simulink model "MotorSimulation"  (R2024b)
settings: Solver=FixedStepAuto  StartTime=0.0  StopTime=5  FixedStep=0.0001  MaxStep=0.001  RelTol=1e-3
model workspace (MAT data in the model file):
  F = 1.3e-07
  J = 1e-09
  K_t = 0.0014172
  L = 0.00024
  R = 2.4
libraries: BrushedDC x1
settings Model: Creator=Daniil  LastModifiedBy=Daniil
settings OptimizationCC: DefaultUnderspecifiedDataType=single
settings RTWCC: BuildConfiguration=Debug  GPUComputeCapability=3.5

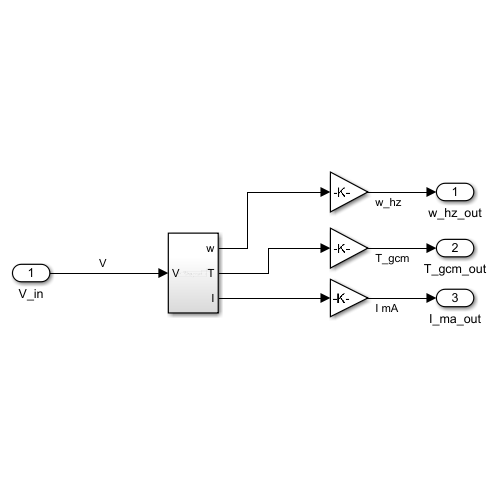
[thumbnail: Simulink's stored preview of the top-level diagram]
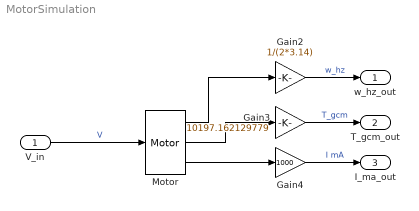
== system MotorSimulation ==
  V_in : Inport
  Gain2 : Gain  Gain=1/(2*3.14)
  Gain3 : Gain  Gain=10197.162129779
  Gain4 : Gain  Gain=1000
  Motor : BrushedDC/Motor  SystemSampleTime=-1  VariantActivationTime=update diagram  AllowFlexibleInterface=on  Latency=0  AutoFrameSizeCalculation=off
  w_hz_out : Outport
  T_gcm_out : Outport  Port=2
  I_ma_out : Outport  Port=3
  wires:
  Gain4/1 -> I_ma_out/1  "I mA"
  Gain3/1 -> T_gcm_out/1  "T_gcm"
  Gain2/1 -> w_hz_out/1  "w_hz"
  V_in/1 -> Motor/1  "V"
  Motor/1 -> Gain2/1
  Motor/2 -> Gain3/1
  Motor/3 -> Gain4/1
